simulink model "PCC_08Jan18_singlephase_actest"  (R2017a)
settings: Solver=ode45  StartTime=0.0  StopTime=.02  RelTol=1e-3  EnableMultiTasking=on
libraries: powerlib x12, powerlib_meascontrol x1, simulink_extras x1
settings Model: Creator=Jawad  LastModifiedBy=Dell
settings DataIOCC: LimitDataPoints=on  SaveFormat=Array  SignalLoggingSaveFormat=ModelDataLogs
settings OptimizationCC: ExpressionDepthLimit=2147483647  LifeSpan=inf
settings DebuggingCC: UnderspecifiedInitializationDetection=Classic  MergeDetectMultiDrivingBlocksExec=none  SolverPrmCheckMsg=warning  FcnCallInpInsideContextMsg=warning  StateNameClashWarn=warning  SFUnexpectedBacktrackingDiag=warning  SFNoUnconditionalDefaultTransitionDiag=warning  SFExecutionAtInitializationDiag=none
settings HardwareCC: ProdBitPerPointer=32  ProdBitPerSizeT=32  ProdBitPerPtrDiffT=32  ProdLargestAtomicFloat=None  ProdIntDivRoundTo=Undefined  ProdEndianess=Unspecified  ProdWordSize=32  ProdHWDeviceType=32-bit Generic
settings ModelReferenceCC: PropagateSignalLabelsOutOfModel=off
settings SFSimCC: SFSimEcho=off
settings GRTTargetCC: TargetLangStandard=C89/C90 (ANSI)  CombineOutputUpdateFcns=off  GRTInterface=on
settings ConfigComp: CovMetricSettings=dw  CovHtmlReporting=on  CovSaveCumulativeToWorkspaceVar=on  CovSaveSingleToWorkspaceVar=on  CovExternalEMLEnable=off

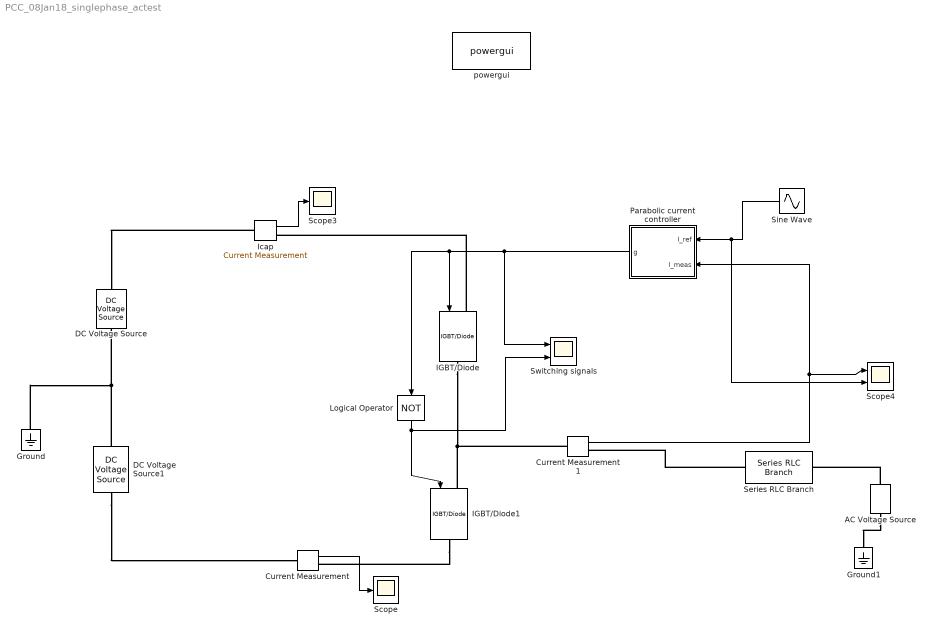
== system PCC_08Jan18_singlephase_actest ==
  AC Voltage Source : powerlib/Electrical Sources/AC Voltage Source  Amplitude=220  Phase=0  Frequency=50  SampleTime=0  Measurements=None  BusType=swing  Pref=10e3  Qref=0  Qmin=-inf  Qmax=+inf
  Current Measurement : powerlib/Measurements/Current Measurement  PhasorSimulation=off  OutputType=Complex  PSBequivalent=0
  Current Measurement1 : powerlib/Measurements/Current Measurement  PhasorSimulation=off  OutputType=Complex  PSBequivalent=0
  DC Voltage Source : powerlib/Electrical Sources/DC Voltage Source  Amplitude=385  Measurements=None
  DC Voltage Source1 : powerlib/Electrical Sources/DC Voltage Source  Amplitude=385  Measurements=None
  Ground : powerlib/Elements/Ground  LConnTagsString=a
  Ground1 : powerlib/Elements/Ground  LConnTagsString=a
  IGBT/Diode : powerlib/Power Electronics/IGBT//Diode  Ron=1e-3  Rs=1e5  Cs=inf  Measurements=off
  IGBT/Diode1 : powerlib/Power Electronics/IGBT//Diode  Ron=1e-3  Rs=1e5  Cs=inf  Measurements=off
  Icap : powerlib/Measurements/Current Measurement  PhasorSimulation=off  OutputType=Complex  PSBequivalent=0
  Logical Operator : Logic  Operator=NOT  AllPortsSameDT=off  OutDataTypeStr=boolean
  Parabolic current controller : Subsystem
  Scope : Scope
  Scope3 : Scope
  Scope4 : Scope  NumInputPorts=2
  Series RLC Branch : powerlib/Elements/Series RLC Branch  LConnTagsString=__new0  RConnTagsString=__new0  BranchType=RL  Resistance=0  Inductance=4e-3  SetiL0=off  InitialCurrent=0  Capacitance=1e-6  Setx0=off  InitialVoltage=0  Measurements=None
  Sine Wave : Sin  Amplitude=9  Frequency=314.16  SampleTime=0
  Switching signals : Scope  NumInputPorts=2
  powergui : powerlib/powergui  Priority=1  SimulationMode=Discrete  SampleTime=5e-7  frequency=60  Iterations=50  frequencyindice=0  Pbase=100e6  ErrMax=1e-4  UnitsV=kV  UnitsW=MW  buscounter=0  FunctionMessages=off  echomessages=off  EnableUseOfTLC=off  CurrentSourceSwitches=off  DisableSnubberDevices=off  DisableRonSwitches=off  DisableVfSwitches=off  DisplayEquations=off  SolverType=Tustin/Backward Euler (TBE)  Interpol=off  ExternalGateDelay=off  methode=off  Ts=0  x0status=blocks  SPID=off  SwTol=0  HookPort=off  RestoreLinks=warning  ResistiveCurrentMeasurement=off  Frange=[0:2:500]  Ylog=off  Xlog=on  ShowGrid=off  save=off  variable=ZData  structure=switching_signal  ZoomFFT=off  StartTime=0.1  cycles=1  DisplayStyle=2  fundamental=50  FreqAxis=on  MaxFrequency=1000  frequencyindicesteady=1  RmsSteady=1  display=off
  wires:
  Current Measurement1/1 -> Parabolic current controller/2(I_meas), Scope4/1
  Parabolic current controller/1(g) -> Switching signals/1, IGBT/Diode/1, Logical Operator/1
  Logical Operator/1 -> IGBT/Diode1/1, Switching signals/2
  Icap/1 -> Scope3/1
  Current Measurement/1 -> Scope/1
  Sine Wave/1 -> Scope4/2, Parabolic current controller/1(I_ref)
  connections:
  DC Voltage Source1/LConn1 -- Current Measurement/LConn1
  Ground/LConn1 -- DC Voltage Source/LConn1 -- DC Voltage Source1/RConn1
  Current Measurement1/LConn1 -- IGBT/Diode/RConn1 -- IGBT/Diode1/LConn1
  Icap/LConn1 -- DC Voltage Source/RConn1
  IGBT/Diode/LConn1 -- Icap/RConn1
  Series RLC Branch/LConn1 -- Current Measurement1/RConn1
  AC Voltage Source/RConn1 -- Series RLC Branch/RConn1
  IGBT/Diode1/RConn1 -- Current Measurement/RConn1
  AC Voltage Source/LConn1 -- Ground1/LConn1

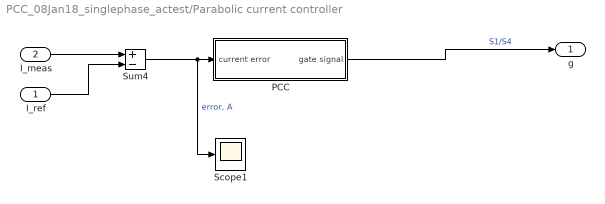
== system PCC_08Jan18_singlephase_actest/Parabolic current controller ==
  I_ref : Inport
  I_meas : Inport  Port=2
  "PCC " : Subsystem
  Scope1 : Scope
  Sum4 : Sum  Inputs=+-
  g : Outport
  wires:
  Sum4/1 -> Scope1/1, "PCC "/1(current error)  "error, A"
  "PCC "/1(gate signal) -> g/1  "S1/S4"
  I_meas/1 -> Sum4/1
  I_ref/1 -> Sum4/2

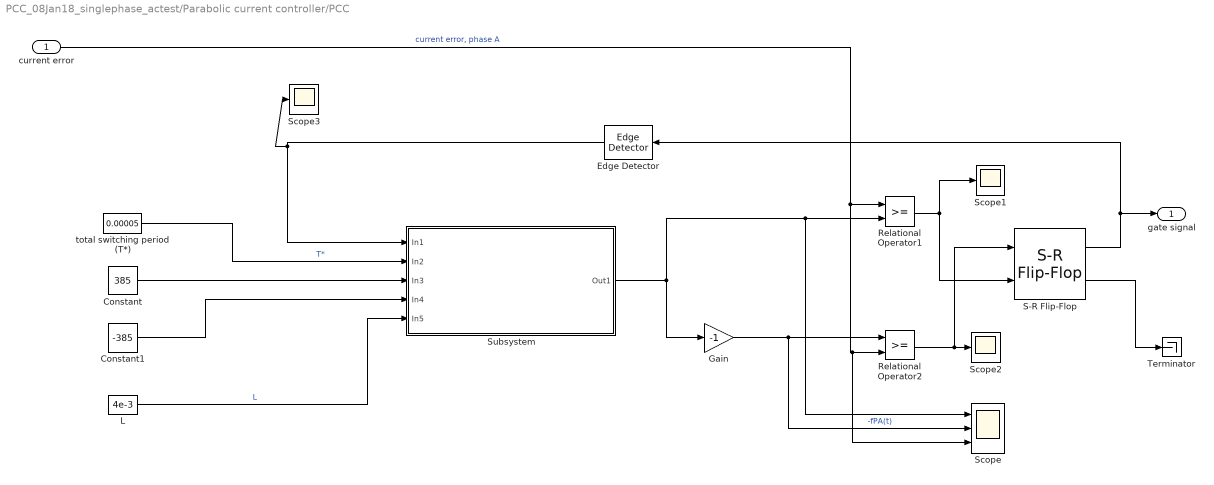
== system PCC_08Jan18_singlephase_actest/Parabolic current controller/PCC  ==
  current error : Inport
  Constant : Constant  Value=385
  Constant1 : Constant  Value=-385
  Edge Detector : powerlib_meascontrol/Logic/Edge Detector  model=Either  ic=0  Ts=0
      settings: SourceProductName=Simscape Power Systems  SourceProductBaseCode=PS
  Gain : Gain  Gain=-1
  L : Constant  Value=4e-3
  Relational Operator1 : RelationalOperator  OutDataTypeStr=boolean  ZeroCross=off  RndMeth=Simplest
  Relational Operator2 : RelationalOperator  OutDataTypeStr=boolean  ZeroCross=off  RndMeth=Simplest
  S-R Flip-Flop : simulink_extras/Flip Flops/S-R Flip-Flop  initial_condition=0
  Scope : Scope  NumInputPorts=3
  Scope1 : Scope
  Scope2 : Scope
  Scope3 : Scope
  Subsystem : Subsystem
  Terminator : Terminator
  total switching period (T*) : Constant  Value=0.00005
  gate signal : Outport
  wires:
  current error/1 -> Relational Operator1/1, Scope/3, Relational Operator2/2  "current error, phase A"
  S-R Flip-Flop/1 -> Edge Detector/1, gate signal/1
  Relational Operator1/1 -> S-R Flip-Flop/2, Scope1/1
  Relational Operator2/1 -> S-R Flip-Flop/1, Scope2/1
  S-R Flip-Flop/2 -> Terminator/1
  Subsystem/1(Out1) -> Gain/1, Scope/1, Relational Operator1/2
  total switching period (T*)/1 -> Subsystem/2(In2)  "T*"
  Constant/1 -> Subsystem/3(In3)
  Constant1/1 -> Subsystem/4(In4)
  L/1 -> Subsystem/5(In5)  "L"
  Gain/1 -> Scope/2, Relational Operator2/1  "-fPA(t)"
  Edge Detector/1 -> Scope3/1, Subsystem/1(In1)

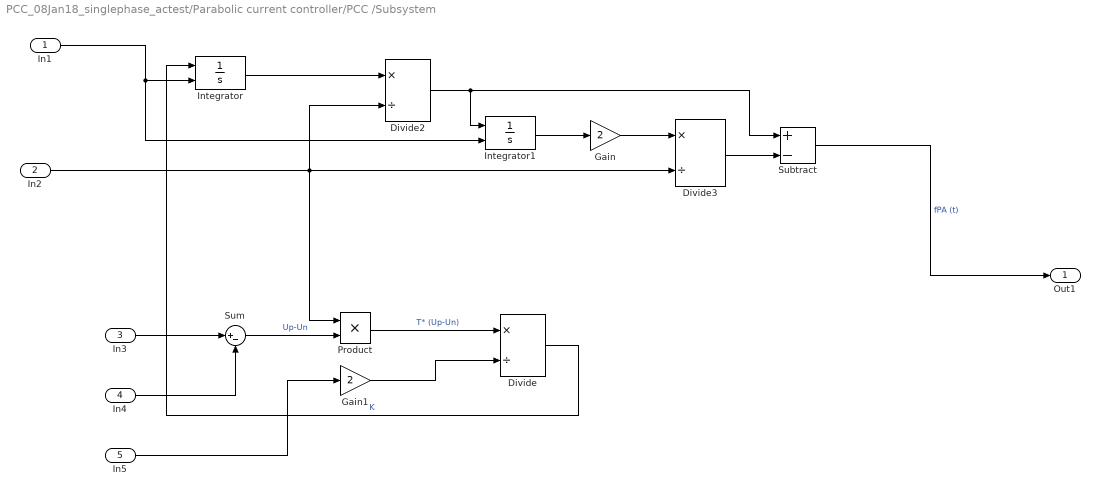
== system PCC_08Jan18_singlephase_actest/Parabolic current controller/PCC /Subsystem ==
  In1 : Inport
  In2 : Inport  Port=2
  In3 : Inport  Port=3
  In4 : Inport  Port=4
  In5 : Inport  Port=5
  Divide : Product  Inputs=*/
  Divide2 : Product  Inputs=*/
  Divide3 : Product  Inputs=*/
  Gain : Gain  Gain=2
  Gain1 : Gain  Gain=2
  Integrator : Integrator  ExternalReset=either
  Integrator1 : Integrator  ExternalReset=either
  Product : Product
  Subtract : Sum  Inputs=+-
  Sum : Sum  Inputs=|+-
  Out1 : Outport
  wires:
  In5/1 -> Gain1/1
  Gain1/1 -> Divide/2
  In3/1 -> Sum/1
  Subtract/1 -> Out1/1  "fPA (t)"
  Sum/1 -> Product/2  "Up-Un"
  In4/1 -> Sum/2
  Product/1 -> Divide/1  "T* (Up-Un)"
  In1/1 -> Integrator1/2, Integrator/2
  Integrator1/1 -> Gain/1
  In2/1 -> Divide3/2, Product/1, Divide2/2
  Divide/1 -> Integrator/1  "K"
  Integrator/1 -> Divide2/1
  Divide2/1 -> Subtract/1, Integrator1/1
  Gain/1 -> Divide3/1
  Divide3/1 -> Subtract/2
